simulink model "dspi_block1130"  (Simulink 8.8)
settings: Solver=FixedStepDiscrete  StartTime=0.0  StopTime=10.0  FixedStep=1  RelTol=1e-3  EnableMultiTasking=on
undefined symbols (not defined in the file or in its folder): A, A14, B, B13, C, CS0, D, D4, F3, F4, G3, G4, H3, H4, K17, K4, L3, N16, N3, P3, PD5, PD6, PD7, R10, R14, R4, SCK, SIN, SOUT, T14
libraries: rappid_564xl_ec_toolbox x12
settings Model: Creator=RMuradov  LastModifiedBy=eugkim01
settings DataIOCC: ExternalInput=off  InitialState=off  SaveOutput=off  SignalLogging=off  SaveTime=off
settings OptimizationCC: DefaultParameterBehavior=Inlined  ExpressionDepthLimit=2147483647  LifeSpan=1
settings DebuggingCC: SolverPrmCheckMsg=warning  InheritedTsInSrcMsg=none  SingleTaskRateTransMsg=error  UnconnectedInputMsg=error  UnconnectedOutputMsg=error  UnconnectedLineMsg=error  UnknownTsInhSupMsg=error
settings HardwareCC: ProdLargestAtomicInteger=Long  ProdLargestAtomicFloat=Double  ProdIntDivRoundTo=Zero  ProdEndianess=BigEndian  ProdHWDeviceType=Freescale->32-bit PowerPC
settings RTWCC: SystemTargetFile=rappid564xl.tlc  MakeCommand=rappid_564xl_make_rtw  TemplateMakefile=rappid_564xl_default_tmf  PostCodeGenCommand=rappid_analyzegencode(buildInfo)  Description=RAppID Toolbox MPC564xL Code Generation Target (rappid)
settings CodeAppCC: IgnoreCustomStorageClasses=off  CustomSymbolStrType=$N$R$M  InternalIdentifier=Classic
settings STFCustomTargetCC: ModelReferenceCompliant=off  CombineOutputUpdateFcns=on  SuppressErrorStatus=on  ERTCustomFileBanners=on  SupportContinuousTime=off  SupportNonInlinedSFcns=off  RemoveResetFunc=on  MATLABClassNameForMDSCustomization=Simulink.SoftwareTarget.ERTCustomization  GRTInterface=off  SystemTargetFile=rappid564xl.tlc
settings ERTTargetCC: MultiwordLength=2048  ModelReferenceCompliant=off  ParMdlRefBuildCompliant=off  CompOptLevelCompliant=off  ConcurrentExecutionCompliant=off  SuppressErrorStatus=on  ERTFirstTimeCompliant=off  ModelStepFunctionPrototypeControlCompliant=off  CPPClassGenCompliant=off  UseToolchainInfoCompliant=off  InlinedParameterPlacement=NonHierarchical  ERTCustomFileTemplate=example_file_process.tlc  ConvertIfToSwitch=off  SuppressUnreachableDefaultCases=off

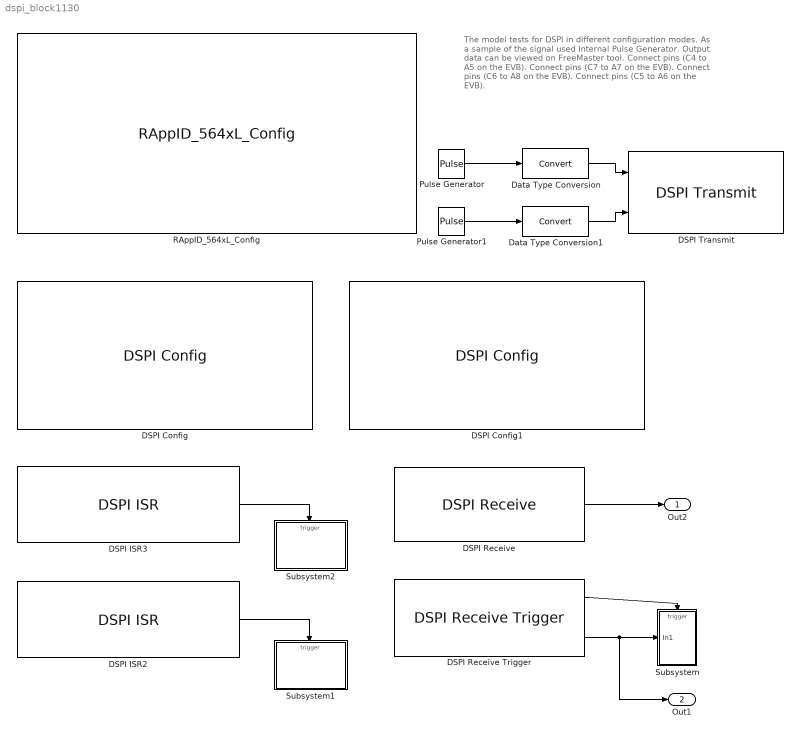
== system dspi_block1130 ==
  note: The model tests for DSPI in different configuration modes.
      |  As a sample of the signal used Internal Pulse Generator.
      | Output data can be viewed on FreeMaster tool.
      |
      | Connect pins (C4 to A5 on the EVB).
      | Connect pins (C7 to A7 on the EVB).
      | Connect pins (C6 to A8 on the EVB).
      | Connect pins (C5 to A6 on the EVB).
  DSPI Config : rappid_564xl_ec_toolbox/MPC564xL/Communication Blocks/DSPI Config  Priority=1  dspi_Num=0  dspi_Mode=Master  dspi_MTFE=off  dspi_CONT_SCKE=off  dspi_PCSSE=off  dspi_ROOE=off  dspi_DIS_TXF=Disable  dspi_DIS_RXF_v2=Disable  dspi_SMPL_PT=DSPI samples SIN at driving SCK edge  dspi_FMSZ=16  dspi_CPOL=Low  dspi_CPHA=Data is captured on the leading edge of SCK and changed on the following edge  dspi_LSBFE=MSB first  dspi_DBR=off  dspi_PCSSCK=1  dspi_PASC=1  dspi_PDT=5  dspi_PBR=5  dspi_CSSCK=256  dspi_ASC=256  dspi_DT=8  dspi_BR=128  dspi_PCSIS0=High  dspi_PCSIS1=High  dspi_PCSIS2=High  dspi_PCSIS3=High  dspi_PCSIS4=High  dspi_PCSIS5=High  dspi_PCSIS6=High  dspi_PCSIS7=High  dspi_DIS_RXF=Oops
  DSPI Config1 : rappid_564xl_ec_toolbox/MPC564xL/Communication Blocks/DSPI Config  Priority=1  dspi_Num=1  dspi_Mode=Slave  dspi_MTFE=off  dspi_CONT_SCKE=off  dspi_PCSSE=off  dspi_ROOE=off  dspi_DIS_TXF=Disable  dspi_DIS_RXF_v2=Disable  dspi_SMPL_PT=DSPI samples SIN at driving SCK edge  dspi_FMSZ=16  dspi_CPOL=Low  dspi_CPHA=Data is captured on the leading edge of SCK and changed on the following edge  dspi_LSBFE=MSB first  dspi_DBR=off  dspi_PCSSCK=1  dspi_PASC=1  dspi_PDT=5  dspi_PBR=5  dspi_CSSCK=256  dspi_ASC=256  dspi_DT=8  dspi_BR=128  dspi_PCSIS0=High  dspi_PCSIS1=High  dspi_PCSIS2=High  dspi_PCSIS3=High  dspi_PCSIS4=High  dspi_PCSIS5=High  dspi_PCSIS6=High  dspi_PCSIS7=High  dspi_DIS_RXF=Oops
  DSPI ISR2 : rappid_564xl_ec_toolbox/MPC564xL/Communication Blocks/DSPI ISR  dspi_Num=0  dspi_isr_name=TCF - Transfer Complete  dspi_isrPrio=14  dspi_isr_tfuf=off  dspi_isr_rfof=on
  DSPI ISR3 : rappid_564xl_ec_toolbox/MPC564xL/Communication Blocks/DSPI ISR  dspi_Num=0  dspi_isr_name=EOQF - End of Queue  dspi_isrPrio=14  dspi_isr_tfuf=off  dspi_isr_rfof=on
  DSPI Receive : rappid_564xl_ec_toolbox/MPC564xL/Communication Blocks/DSPI Receive  dspi_Num=0
  DSPI Receive Trigger : rappid_564xl_ec_toolbox/MPC564xL/Communication Blocks/DSPI Receive Trigger  dspi_Num=1  dspi_ISRPri=13
  DSPI Transmit : rappid_564xl_ec_toolbox/MPC564xL/Communication Blocks/DSPI Transmit  Priority=2  dspi_Num=0  dspi_CONT=off  dspi_PUSHR_PE=off  dspi_PUSHR_PP=off  dspi_PCS_0=36 : C[4] : [11] : [H3] : CS0  dspi_PCS_1=5 : A[5] : [14] : [H4] : CS0  dspi_PCS_2=3 : A[3] : [92] : [K17] : CS0  dspi_PCS_slave_0=36 : C[4] : [11] : [H3] : CS0  dspi_PCS_slave_1=5 : A[5] : [14] : [H4] : CS0  dspi_PCS_slave_2=3 : A[3] : [92] : [K17] : CS0  dspi_SIN_0=39 : C[7] : [15] : [K4] : SIN  dspi_SIN_1=8 : A[8] : [12] : [F4]  dspi_SIN_2=2 : A[2] : [84] : [N16] : SIN  dspi_SCK_0=37 : C[5] : [13] : [G3] : SCK  dspi_SCK_1=6 : A[6] : [2] : [G4] : SCK  dspi_SCK_2=0 : A[0] : [73] : [T14] : SCK  dspi_SOUT_0=38 : C[6] : [142] : [D4] : SOUT  dspi_SOUT_1=7 : A[7] : [10] : [F3] : SOUT  dspi_SOUT_2=1 : A[1] : [74] : [R14] : SOUT  dspi_Strobe=None  dspi_eoq=on  dspi_pcsx=Assert
  Data Type Conversion : DataTypeConversion  Priority=1
  Data Type Conversion1 : DataTypeConversion  Priority=1
  Pulse Generator : DiscretePulseGenerator  Amplitude=85
  Pulse Generator1 : DiscretePulseGenerator  Period=5  PulseWidth=3
  RAppID_564xL_Config : rappid_564xl_ec_toolbox/MPC564xL/RAppID_564xL_Config  SystemClock=120  XTAL=40  MC_clock_60=12  MC_clock_80=16  MC_clock_120=10  SWG_clock_60=20  SWG_clock_80=13.334  SWG_clock_120=20  Compiler=CodeWarrior  MemTarget=RAM  Part=MPC5643L  Package=144 LQFP  global_int_priority=0  base_tick_priority=10  sys_task_supress=off  exception_handlers=off  stored_mdl_name=dspi_block_temp  freemaster_interface=Oops  freemaster_rx_pin="LINFlex_0 Rx Pin 116 : \"PB[3]\""  freemaster_tx_pin="LINFlex_0 Tx Pin 114 : \"PB[2]\""  freemaster_interface_1=Serial 0  freemaster_enable=on  freemaster_rate=57600  freemaster_tx0_pin=18 : B[2] : 114 : A14  freemaster_rx0_pin=19 : B[3] : 116 : B13  freemaster_tx1_pin=57 : D[9] : 26 : L3  freemaster_rx1_pin=29 : B[13] : 60 : R10  freemaster_can_channel=1CH  freemater_can_speed=500K  freemaster_can_msgig=0x7AA  ccp_interface=None  ccp_enable=off  ccp_can_channel=CH1 (MB 0 - 1)  ccp_can_speed=500K  ccp_can_cro_id=256  ccp_can_dto_id=257  ccp_dev_id=RappID  ccp_dev_addr=0  ccp_odt=3  ccp_daq=3  pil_enable=off  pil_bam=on  comport=6  pil_rate=57600  bam_password_def=on  bam_password=0xFEEDFACECAFEBEEF  bam_sa_cs=off  bam_start_address=0x0  bam_code_size=0x7000  cons_dspi=on  cons_can=on  cons_adc=on  cons_pwm=on  cons_ctu=on  cons_swg=on  cons_eTimer=on  cons_fm=on
  Subsystem : Subsystem
      settings: RTWSystemCode=Nonreusable function
  Subsystem1 : Subsystem
      settings: RTWSystemCode=Nonreusable function
  Subsystem2 : Subsystem
      settings: RTWSystemCode=Nonreusable function
  Out2 : Outport
  Out1 : Outport  Port=2
  wires:
  Pulse Generator/1 -> Data Type Conversion/1
  Data Type Conversion/1 -> DSPI Transmit/1
  DSPI Receive/1 -> Out2/1
  DSPI Receive Trigger/2 -> Subsystem/1(In1), Out1/1
  DSPI Receive Trigger/1 -> Subsystem/Trigger
  DSPI ISR2/1 -> Subsystem1/Trigger
  Pulse Generator1/1 -> Data Type Conversion1/1
  Data Type Conversion1/1 -> DSPI Transmit/2
  DSPI ISR3/1 -> Subsystem2/Trigger

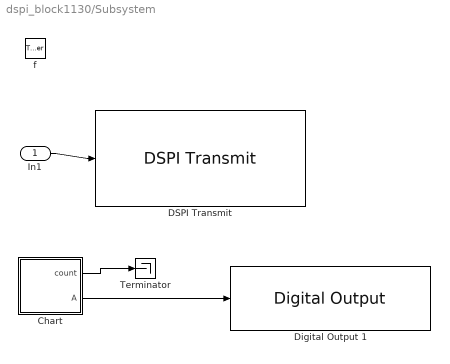
== system dspi_block1130/Subsystem ==
  In1 : Inport
  f : TriggerPort  TriggerType=function-call  VariantControl=Variant
  Chart : Stateflow chart  TreatAsAtomicUnit=on
  DSPI Transmit : rappid_564xl_ec_toolbox/MPC564xL/Communication Blocks/DSPI Transmit  Priority=2  dspi_Num=1  dspi_CONT=off  dspi_PUSHR_PE=off  dspi_PUSHR_PP=off  dspi_PCS_0=36 : C[4] : [11] : [H3] : CS0  dspi_PCS_1=5 : A[5] : [14] : [H4] : CS0  dspi_PCS_2=3 : A[3] : [92] : [K17] : CS0  dspi_PCS_slave_0=36 : C[4] : [11] : [H3] : CS0  dspi_PCS_slave_1=5 : A[5] : [14] : [H4] : CS0  dspi_PCS_slave_2=3 : A[3] : [92] : [K17] : CS0  dspi_SIN_0=39 : C[7] : [15] : [K4] : SIN  dspi_SIN_1=8 : A[8] : [12] : [F4]  dspi_SIN_2=2 : A[2] : [84] : [N16] : SIN  dspi_SCK_0=37 : C[5] : [13] : [G3] : SCK  dspi_SCK_1=6 : A[6] : [2] : [G4] : SCK  dspi_SCK_2=0 : A[0] : [73] : [T14] : SCK  dspi_SOUT_0=38 : C[6] : [142] : [D4] : SOUT  dspi_SOUT_1=7 : A[7] : [10] : [F3] : SOUT  dspi_SOUT_2=1 : A[1] : [74] : [R14] : SOUT  dspi_Strobe=None  dspi_eoq=off  dspi_pcsx=Assert
  Digital Output 1 : rappid_564xl_ec_toolbox/MPC564xL/General Purpose Blocks/Digital Output   gpio_outputs="55  : PD7  : [ 37 ] : [ R4 ]"  pinNum=[ 37 ]  pcrNum=55
  Terminator : Terminator
  wires:
  In1/1 -> DSPI Transmit/1
  Chart/1(count) -> Terminator/1
  Chart/2(" A") -> Digital Output 1/1

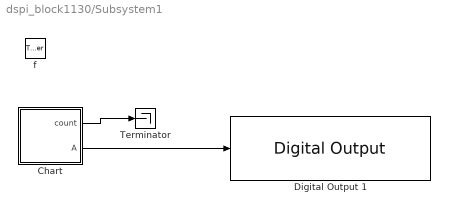
== system dspi_block1130/Subsystem1 ==
  f : TriggerPort  TriggerType=function-call  VariantControl=Variant
  Chart : Stateflow chart  TreatAsAtomicUnit=on
  Digital Output 1 : rappid_564xl_ec_toolbox/MPC564xL/General Purpose Blocks/Digital Output   gpio_outputs="53  : PD5  : [ 33 ] : [ N3 ]"  pinNum=[ 33 ]  pcrNum=53
  Terminator : Terminator
  wires:
  Chart/1(count) -> Terminator/1
  Chart/2(" A") -> Digital Output 1/1

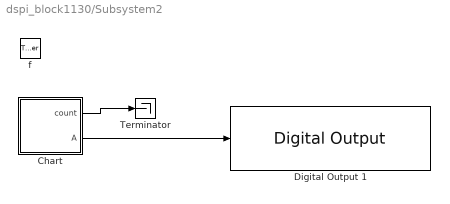
== system dspi_block1130/Subsystem2 ==
  f : TriggerPort  TriggerType=function-call  VariantControl=Variant
  Chart : Stateflow chart  TreatAsAtomicUnit=on
  Digital Output 1 : rappid_564xl_ec_toolbox/MPC564xL/General Purpose Blocks/Digital Output   gpio_outputs="54  : PD6  : [ 34 ] : [ P3 ]"  pinNum=[ 34 ]  pcrNum=54
  Terminator : Terminator
  wires:
  Chart/1(count) -> Terminator/1
  Chart/2(" A") -> Digital Output 1/1

== stateflow chart Subsystem2/Chart ==
  state A
  state A1
  (default) -> A : {count =0;}
  A -> A1
  A1 -> A : { count = count + 1;}
  data: count output double; A output boolean

== stateflow chart Subsystem/Chart ==
  state A
  state A1
  (default) -> A : {count =0;}
  A -> A1
  A1 -> A : { count = count + 1;}
  data: count output double; A output boolean

== stateflow chart Subsystem1/Chart ==
  state A
  state A1
  (default) -> A : {count =0;}
  A -> A1
  A1 -> A : { count = count + 1;}
  data: count output double; A output boolean
